simulink model "prob3"  (Simulink 8.9)
settings: Solver=ode45  StartTime=0.0  StopTime=80  RelTol=1e-3  EnableMultiTasking=on
values from neighbouring files (symbols this model uses):
  delta_e_max = 30 * pi / 180    (= 0.523598775598)    [parameters.m]
  kd_th = (2 * zeta_th * omega_n_th - ath1) / ath3    [parameters.m]
  ki_h = omega_n_h ^ 2 / (Kdc_th * ah1)    [parameters.m]
  kp_h = 2 * zeta_h * omega_n_h / (Kdc_th * ah1)    [parameters.m]
  kp_th = -delta_e_max / th_max    (= -3)    [parameters.m]
settings Model: SuppressorTable=22 serialization::archive 11 0 6 0 0 0 11 0  Creator=tmclain  LastModifiedBy=erichm
settings DataIOCC: SignalLoggingSaveFormat=Dataset
settings OptimizationCC: ExpressionDepthLimit=2147483647
settings DebuggingCC: SolverPrmCheckMsg=warning  FcnCallInpInsideContextMsg=error
settings GRTTargetCC: CombineOutputUpdateFcns=on  GRTInterface=off

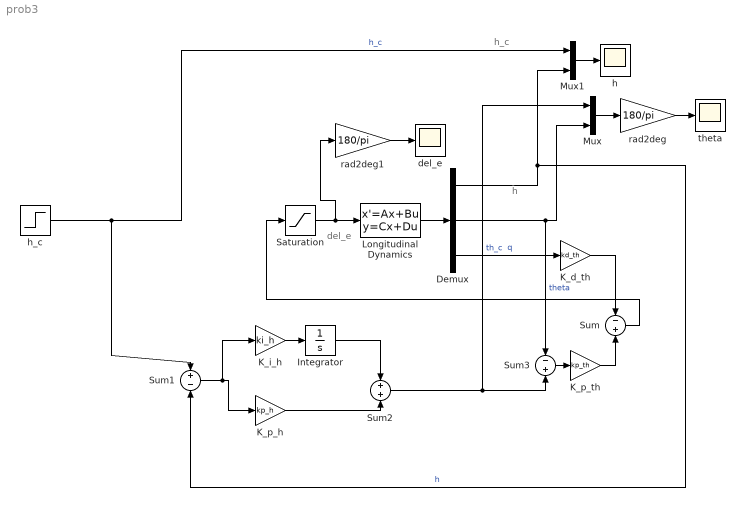
== system prob3 ==
  note: del_e
  note: h_c
  note: h
  Demux : Demux  Outputs=3
  Integrator : Integrator
  K_d_th : Gain  Gain=kd_th
  K_i_h : Gain  Gain=ki_h
  K_p_h : Gain  Gain=kp_h
  K_p_th : Gain  Gain=kp_th
  Longitudinal Dynamics : StateSpace  A=[-0.00643 0.0263 0 -32.2 0; -0.0941 -0.624 820 0 0; -0.000222 -0.00153 -0.668 0 0; 0 0 1 0 0; 0 -1 0 830 0]  B=[0; -32.7; -2.08; 0; 0]  C=[0 0 0 0 1; 0 0 0 1 0; 0 0 1 0 0]  D=[0; 0; 0]  X0=0
  Mux : Mux  Inputs=2
  Mux1 : Mux  Inputs=2
  Saturation : Saturate  UpperLimit=delta_e_max  LowerLimit=-delta_e_max
  Sum : Sum  Inputs=-+
  Sum1 : Sum  Inputs=+-
  Sum2 : Sum
  Sum3 : Sum  Inputs=-+
  del_e : Scope
  h : Scope
  "h_c " : Step  Time=10  After=100  SampleTime=0
  rad2deg : Gain  Gain=180/pi
  rad2deg1 : Gain  Gain=180/pi
  theta : Scope
  wires:
  Longitudinal Dynamics/1 -> Demux/1
  Demux/1 -> Sum1/2, Mux1/2  "h"
  Demux/2 -> Sum3/1, Mux/2  "theta"
  rad2deg/1 -> theta/1
  Mux/1 -> rad2deg/1
  Mux1/1 -> h/1
  rad2deg1/1 -> del_e/1
  "h_c "/1 -> Sum1/1, Mux1/1  "h_c"
  Demux/3 -> K_d_th/1  "q"
  Saturation/1 -> rad2deg1/1, Longitudinal Dynamics/1
  K_d_th/1 -> Sum/1
  K_p_th/1 -> Sum/2
  Sum/1 -> Saturation/1
  K_i_h/1 -> Integrator/1
  Sum1/1 -> K_i_h/1, K_p_h/1
  K_p_h/1 -> Sum2/2
  Integrator/1 -> Sum2/1
  Sum2/1 -> Mux/1, Sum3/2  "th_c"
  Sum3/1 -> K_p_th/1
